simulink model "Actuators"  (Simulink 8.4)
settings: Solver=ode45  StartTime=0.0  StopTime=10.0  RelTol=1e-3
undefined symbols (not defined in the file): Ais_flgAirInjReacPumpOverride, Ais_stAirInjReacPumpMan, Apv_facAirPumpRateMan, Apv_factor, Apv_flgAirPumpRateOverride, Apv_tiPeriod_C, CDRV_E_OK_, Cov_facChOverVlvRateMan, Cov_factor, Cov_flgChOverVlvRateOverride, Cov_tiPeriod_C, Doh_OutputDiagnosisOverride, Fps_flgFuelPumpOverride, Fps_stFuelPumpMan, Icc_degIgnMan, Icc_flgIgnAngleOverride, Icc_flgIgnCutoffMan, Icc_flgIgnCutoffOverride, Icc_nrFollowUpSparks, Icc_tiDwell, Icc_tiDwellFollowUpSparks, Icc_tiOffFollowUpSparks, Ics_flgIntercoolerOverride, Ics_stIntercoolerMan, Ivc_degInjAbort, Ivc_degIntakeClose, Ivc_degOffsetInjEndSimultanInj, Ivc_flgBattDelayOverride, Ivc_flgDiagEntryCondFulfilled, Ivc_flgEndOfStartCond, Ivc_flgInjCutoff, Ivc_flgInjCutoffOverride, Ivc_flgInjTimeOverride, Ivc_flgOverrunCutoff, Ivc_flgPostInjCond, Ivc_tiBattDelayMan, Ivc_tiInjEff, Ivc_tiInjMan, Ivc_tiMinThresDeltaEffInjPeriod, Ivc_weea0, Ivc_weea1, Ivc_weea2, Lo_, Mrs_flgMainRelaisOverride, Mrs_stMainRelaisMan, Normal, OK, OpenCircuit, OverTemp, ShortToBatt, ShortToBattNEG, ShortToGnd, ShortToGndNEG, ShortToGndPOS, Str_flgStarterOverride, Str_stStarterMan, Tvc_facDutycyclePIDLimitMax, Tvc_facDutycyclePIDLimitMin, Tvc_facDutycyclePilotControlNeg, Tvc_facDutycyclePilotControlPos ... (+20)
libraries: simulink x9
(part 3 of 3)

== system Actuators/Actuators_mdl/Mrs/G1_DigOut_GetError ==
  DTC_DigOut_GetError : DataTypeConversion  OutDataTypeStr=single
  FlexECU_DevLib_FcnAPI_Wrapper_SFcn : S-Function  FunctionName=ehooks_medc17flex_devlib_basic_io_fcncall  Parameters=NoInputPorts, NoOutputPorts, InputPortDataTypes, OutputPortDataTypes, CFunctionArgTypes, CFunctionName, ChannelName  EnableBusSupport=off  mask{NoInputPorts=0, NoOutputPorts=1, InputPortDataTypes=, OutputPortDataTypes=uint8, CFunctionArgTypes=ret, CFunctionName=DevLib_DioSet_GetError, ChannelName=O_S_MRLY}
      mask prompts: NoInputPorts "Number of input ports"; NoOutputPorts "Number of output ports"; InputPortDataTypes "Input port data types"; OutputPortDataTypes "Output port data types"; CFunctionArgTypes "C function argument types"; CFunctionName "C function name"; ChannelName "Channel (pin) name"
      mask Display: disp('EHOOKS FlexECU\nDevLib Wrapper\nS-Function')
  status : Outport
  wires:
  DTC_DigOut_GetError/1 -> status/1
  FlexECU_DevLib_FcnAPI_Wrapper_SFcn/1 -> DTC_DigOut_GetError/1

== system Actuators/Actuators_mdl/Str/G1_DigOut_Ctrl ==
  state : Inport
  DTC_DigOut_ctrl : DataTypeConversion  OutDataTypeStr=uint8  RndMeth=Nearest
  DTC_Out1 : DataTypeConversion  OutDataTypeStr=boolean
  FlexECU_DevLib_FcnAPI_Wrapper_SFcn : S-Function  FunctionName=ehooks_medc17flex_devlib_basic_io_fcncall  Parameters=NoInputPorts, NoOutputPorts, InputPortDataTypes, OutputPortDataTypes, CFunctionArgTypes, CFunctionName, ChannelName  EnableBusSupport=off  mask{NoInputPorts=1, NoOutputPorts=1, InputPortDataTypes=uint8, OutputPortDataTypes=uint8, CFunctionArgTypes=ret,val, CFunctionName=DevLib_Dio_Set, ChannelName=O_S_RL34}
      mask prompts: NoInputPorts "Number of input ports"; NoOutputPorts "Number of output ports"; InputPortDataTypes "Input port data types"; OutputPortDataTypes "Output port data types"; CFunctionArgTypes "C function argument types"; CFunctionName "C function name"; ChannelName "Channel (pin) name"
      mask Display: disp('EHOOKS FlexECU\nDevLib Wrapper\nS-Function')
  status : Outport
  wires:
  DTC_DigOut_ctrl/1 -> FlexECU_DevLib_FcnAPI_Wrapper_SFcn/1
  state/1 -> DTC_DigOut_ctrl/1
  FlexECU_DevLib_FcnAPI_Wrapper_SFcn/1 -> DTC_Out1/1
  DTC_Out1/1 -> status/1

== system Actuators/Actuators_mdl/Str/G1_DigOut_GetError ==
  DTC_DigOut_GetError : DataTypeConversion  OutDataTypeStr=single
  FlexECU_DevLib_FcnAPI_Wrapper_SFcn : S-Function  FunctionName=ehooks_medc17flex_devlib_basic_io_fcncall  Parameters=NoInputPorts, NoOutputPorts, InputPortDataTypes, OutputPortDataTypes, CFunctionArgTypes, CFunctionName, ChannelName  EnableBusSupport=off  mask{NoInputPorts=0, NoOutputPorts=1, InputPortDataTypes=, OutputPortDataTypes=uint8, CFunctionArgTypes=ret, CFunctionName=DevLib_DioSet_GetError, ChannelName=O_S_RL34}
      mask prompts: NoInputPorts "Number of input ports"; NoOutputPorts "Number of output ports"; InputPortDataTypes "Input port data types"; OutputPortDataTypes "Output port data types"; CFunctionArgTypes "C function argument types"; CFunctionName "C function name"; ChannelName "Channel (pin) name"
      mask Display: disp('EHOOKS FlexECU\nDevLib Wrapper\nS-Function')
  status : Outport
  wires:
  DTC_DigOut_GetError/1 -> status/1
  FlexECU_DevLib_FcnAPI_Wrapper_SFcn/1 -> DTC_DigOut_GetError/1

== system Actuators/Actuators_mdl/Tvc/Limiter ==
  max : Inport
  in : Inport  Port=2
  min : Inport  Port=3
  Saturation Dynamic : simulink/Discontinuities/Saturation Dynamic  OutMin=[]  OutMax=[]  OutDataTypeStr=Inherit: Same as second input  OutDataType=fixdt(1, 16)  OutScaling=2^-10  DoSatur=off
  return : Outport
  wires:
  max/1 -> Saturation Dynamic/1
  in/1 -> Saturation Dynamic/2
  min/1 -> Saturation Dynamic/3
  Saturation Dynamic/1 -> return/1

== system Actuators/Actuators_mdl/Tvc/ThrottleValveControl ==
  Tvc_flgPosError : Inport
  Tvc_facThrValve : Inport  Port=2
  Tvc_facThrValveReq : Inport  Port=3
  Add : Sum  OutDataTypeStr=Inherit: Same as first input
  Constan1 : Constant  Value=0.0  OutDataTypeStr=single
  Constan2 : Constant  Value=0.01  OutDataTypeStr=single
  Constant1 : Constant  Value=Tvc_facDutycyclePilotControlPos  OutDataTypeStr=single
  Constant2 : Constant  Value=Tvc_facDutycyclePilotControlNeg  OutDataTypeStr=single
  Constant3 : Constant  Value=Tvc_flgThrValveDutycycleOverride
  Constant4 : Constant  Value=Tvc_facThrValveDutycycleMan
  Constant5 : Constant  Value=Tvc_tiTnDutycycle
  Constant6 : Constant  Value=Tvc_tiTvDutycycle
  Constant7 : Constant  Value=Tvc_facKDutycycle
  Constant8 : Constant  Value=Tvc_facDutycyclePIDLimitMax
  Constant9 : Constant  Value=Tvc_facDutycyclePIDLimitMin
  Logical Operator1 : Logic  Operator=NOT  AllPortsSameDT=off  OutDataTypeStr=boolean
  Manual Switch : ManualSwitch
  PID_Limit_AWU : Subsystem
      mask help: PID_Limit_AWU
      mask Display: image(imread('PID_Limit_AWU.jpg'))
  PID_Limit_AWU_Fcn : Subsystem
      mask help: PID_Limit_AWU_Fcn
      mask Display: image(imread('PID_Limit_AWU.jpg'))
  Relational Operator : RelationalOperator  Operator=<  OutDataTypeStr=boolean
  Subtract : Sum  Inputs=+-  OutDataTypeStr=Inherit: Same as first input
  Switch : Switch  Threshold=1
  Switch1 : Switch  Threshold=1
  Tvc_facDutycycle : Outport
  wires:
  Constant3/1 -> Switch1/2
  Constant4/1 -> Switch1/1
  Add/1 -> Switch1/3
  Constan1/1 -> Relational Operator/2
  Relational Operator/1 -> Switch/2
  Switch/1 -> Add/1
  Switch1/1 -> Tvc_facDutycycle/1
  Tvc_flgPosError/1 -> Logical Operator1/1
  Constant5/1 -> PID_Limit_AWU/1(Tn)
  Constan2/1 -> PID_Limit_AWU/3(Ta)
  Subtract/1 -> PID_Limit_AWU/5(in), PID_Limit_AWU_Fcn/1(in)
  Constant6/1 -> PID_Limit_AWU/2(Tv)
  Constant7/1 -> PID_Limit_AWU/4(Kp)
  Tvc_facThrValveReq/1 -> Subtract/2
  Tvc_facThrValve/1 -> Subtract/1, Relational Operator/1
  Constant2/1 -> Switch/1
  Constant1/1 -> Switch/3
  Logical Operator1/1 -> PID_Limit_AWU_Fcn/2(initValue), PID_Limit_AWU/6(initValue)
  Constant8/1 -> PID_Limit_AWU/7(outMax)
  Constant9/1 -> PID_Limit_AWU/8(outMin)
  PID_Limit_AWU_Fcn/1(Tvc_facDutycycleCorr) -> Manual Switch/2  "Tvc_facDutycycleCorr_Fcn"
  PID_Limit_AWU/1(Tvc_facDutycycleCorr) -> Manual Switch/1  "Tvc_facDutycycleCorr"
  Manual Switch/1 -> Add/2

== system Actuators/Actuators_mdl/Tvc/ThrottleValveOutput ==
  Tvc_flgPosError : Inport
  Tvc_facDutycycle : Inport  Port=2
  Constant1 : Constant  Value=Tvc_tiPeriod_C
  Constant3 : Constant  Value=Lo_
  Constant5 : Constant  Value=Normal
  G1_HbridgeOut_Ctrl : Subsystem  AncestorBlock=ehooks_medc17flex_G1_lib/Library Blocks/Basic_IO/Outputs/G1_HbridgeOut_Ctrl  mask{ChannelName=O_T_DC1}
      mask prompts: ChannelName "Channel name"
      mask init:
      | ehooks_medc17flex_devlib_io_block('mask_init');
      settings: AttributesFormatString=Channel name: '%<ChannelName>'
      mask TypeOptions ChannelName: <empty> | O_T_DC1 | O_T_DC2 | O_T_DC3
      mask Display: image(imread('Output_HBridge.jpg'))
  G1_Hbridge_Get_error : Subsystem  AncestorBlock=ehooks_medc17flex_G1_lib/Library Blocks/Basic_IO/Outputs/G1_Hbridge_Get_error  mask{ChannelName=O_T_DC1}
      mask prompts: ChannelName "Channel name"
      mask init:
      | ehooks_medc17flex_devlib_io_block('mask_init');
      settings: AttributesFormatString=Channel name: '%<ChannelName>'
      mask TypeOptions ChannelName: <empty> | O_T_DC1 | O_T_DC2 | O_T_DC3
      mask Display: image(imread('Output_HBridge_Diagnosis.jpg'))
  Interval Test : simulink/Logic and Bit Operations/Interval Test  IntervalClosedRight=on  uplimit=1  IntervalClosedLeft=on  lowlimit=-1  OutDataTypeStr=boolean
  Logical Operator : Logic  Operator=OR  Inputs=3  AllPortsSameDT=off  OutDataTypeStr=boolean
  Relational Operator : RelationalOperator  Operator=~=  OutDataTypeStr=boolean
  Tvc_stHBridge : Outport
  Tvc_stDiagnosis : Outport  Port=2
  wires:
  Constant1/1 -> G1_HbridgeOut_Ctrl/3(period)
  Tvc_facDutycycle/1 -> G1_HbridgeOut_Ctrl/1(dutycycle), Interval Test/1
  G1_HbridgeOut_Ctrl/1(status) -> Tvc_stHBridge/1
  Logical Operator/1 -> G1_HbridgeOut_Ctrl/2(disable)
  Interval Test/1 -> Logical Operator/1
  Constant3/1 -> G1_HbridgeOut_Ctrl/4(level)
  G1_Hbridge_Get_error/1(status) -> Tvc_stDiagnosis/1
  [Opm_idxMode_global] -> Relational Operator/1
  Constant5/1 -> Relational Operator/2
  Tvc_flgPosError/1 -> Logical Operator/2
  Relational Operator/1 -> Logical Operator/3

== system Actuators/Actuators_mdl/Tvc/ThrottleValvePosition ==
  Abs : Abs
  Add : Sum  OutDataTypeStr=Inherit: Same as first input
  Constan1 : Constant  Value=0.05  OutDataTypeStr=single
  Constant : Constant  Value=2  OutDataTypeStr=single
  Divide : Product  Inputs=*/  OutDataTypeStr=Inherit: Same as first input
  G1_ADC_Input_Receive : Subsystem  AncestorBlock=ehooks_medc17flex_G1_lib/Library Blocks/Basic_IO/Inputs/G1_ADC_Input_Receive  mask{ChannelName=I_A_AN01}
      mask prompts: ChannelName "Channel name"
      mask init:
      | ehooks_medc17flex_devlib_io_block('mask_init');
      settings: AttributesFormatString=Channel name: '%<ChannelName>'
      mask TypeOptions ChannelName: <empty> | I_A_AN01 | I_A_AN02 | I_A_AN03 | I_A_AN05 | I_A_AN06 | I_A_AN07 | I_A_AN08 | I_A_AN10 | I_A_AN11 | I_A_AN12 | I_A_AN13 | I_A_AN14 | I_A_AN15 | I_A_AN16 | I_A_AN17 | I_A_AN18 | I_A_AN19 | I_A_AN20 | I_A_AN21 | I_A_AN23 | I_A_AN32 | I_A_AN35 | I_A_AN36 | I_A_AN37 | I_A_AN39 | I_A_AN100 | I_A_AN101 | I_A_AN103 | I_A_AN104 | I_A_AN105 | I_A_AN106
      mask Display: image(imread('Input_Analog.jpg'))
  G1_ADC_Input_Receive1 : Subsystem  AncestorBlock=ehooks_medc17flex_G1_lib/Library Blocks/Basic_IO/Inputs/G1_ADC_Input_Receive  mask{ChannelName=I_A_AN02}
      mask prompts: ChannelName "Channel name"
      mask init:
      | ehooks_medc17flex_devlib_io_block('mask_init');
      settings: AttributesFormatString=Channel name: '%<ChannelName>'
      mask TypeOptions ChannelName: <empty> | I_A_AN01 | I_A_AN02 | I_A_AN03 | I_A_AN05 | I_A_AN06 | I_A_AN07 | I_A_AN08 | I_A_AN10 | I_A_AN11 | I_A_AN12 | I_A_AN13 | I_A_AN14 | I_A_AN15 | I_A_AN16 | I_A_AN17 | I_A_AN18 | I_A_AN19 | I_A_AN20 | I_A_AN21 | I_A_AN23 | I_A_AN32 | I_A_AN35 | I_A_AN36 | I_A_AN37 | I_A_AN39 | I_A_AN100 | I_A_AN101 | I_A_AN103 | I_A_AN104 | I_A_AN105 | I_A_AN106
      mask Display: image(imread('Input_Analog.jpg'))
  Interval Test : simulink/Logic and Bit Operations/Interval Test  IntervalClosedRight=on  uplimit=Tvc_uSensMaxValid  IntervalClosedLeft=on  lowlimit=Tvc_uSensMinValid  OutDataTypeStr=boolean
  Interval Test1 : simulink/Logic and Bit Operations/Interval Test  IntervalClosedRight=on  uplimit=Tvc_uSensMaxValid  IntervalClosedLeft=on  lowlimit=Tvc_uSensMinValid  OutDataTypeStr=boolean
  Logical Operator{,1..3} (4 alike) : Logic  Operator=NOT  AllPortsSameDT=off  OutDataTypeStr=boolean
  Logical Operator4 : Logic  Operator=OR  Inputs=5  AllPortsSameDT=off  OutDataTypeStr=boolean
  Relational Oprator : RelationalOperator  Operator=>  OutDataTypeStr=boolean
  Subtract : Sum  Inputs=+-  OutDataTypeStr=Inherit: Same as first input
  Tvc_uSens2facThrValve1_CUR : Lookup_n-D  NumberOfTableDimensions=1  BreakpointsForDimension1=[1:3]  Table=[1 3 6]  ExtrapMethod=Clip  OutDataTypeStr=Inherit: Inherit from 'Table data'  InputSameDT=on
  Tvc_uSens2facThrValve2_CUR : Lookup_n-D  NumberOfTableDimensions=1  BreakpointsForDimension1=[1:3]  Table=[1 2 7]  ExtrapMethod=Clip  OutDataTypeStr=Inherit: Inherit from 'Table data'  InputSameDT=on
  Tvc_flgPosError : Outport
  Tvc_facThrValve : Outport  Port=2
  wires:
  G1_ADC_Input_Receive/1(status) -> Logical Operator/1  "Tvc_stIO1"
  G1_ADC_Input_Receive/2(uRaw) -> Tvc_uSens2facThrValve1_CUR/1, Interval Test/1  "Tvc_uSens1"
  G1_ADC_Input_Receive1/1(status) -> Logical Operator2/1  "Tvc_stIO2"
  G1_ADC_Input_Receive1/2(uRaw) -> Tvc_uSens2facThrValve2_CUR/1, Interval Test1/1  "Tvc_uSens2"
  Interval Test/1 -> Logical Operator1/1
  Interval Test1/1 -> Logical Operator3/1
  Tvc_uSens2facThrValve1_CUR/1 -> Add/1, Subtract/1  "Tvc_facThrValve1"
  Tvc_uSens2facThrValve2_CUR/1 -> Add/2, Subtract/2  "Tvc_facThrValve2"
  Add/1 -> Divide/1
  Constant/1 -> Divide/2
  Subtract/1 -> Abs/1
  Abs/1 -> Relational Oprator/1
  Constan1/1 -> Relational Oprator/2
  Logical Operator4/1 -> Tvc_flgPosError/1
  Logical Operator/1 -> Logical Operator4/1
  Logical Operator1/1 -> Logical Operator4/2
  Logical Operator2/1 -> Logical Operator4/3
  Logical Operator3/1 -> Logical Operator4/4
  Relational Oprator/1 -> Logical Operator4/5
  Divide/1 -> Tvc_facThrValve/1

== system Actuators/Actuators_mdl/Wcs/G1_DigOut_Ctrl ==
  state : Inport
  DTC_DigOut_ctrl : DataTypeConversion  OutDataTypeStr=uint8  RndMeth=Nearest
  DTC_Out1 : DataTypeConversion  OutDataTypeStr=boolean
  FlexECU_DevLib_FcnAPI_Wrapper_SFcn : S-Function  FunctionName=ehooks_medc17flex_devlib_basic_io_fcncall  Parameters=NoInputPorts, NoOutputPorts, InputPortDataTypes, OutputPortDataTypes, CFunctionArgTypes, CFunctionName, ChannelName  EnableBusSupport=off  mask{NoInputPorts=1, NoOutputPorts=1, InputPortDataTypes=uint8, OutputPortDataTypes=uint8, CFunctionArgTypes=ret,val, CFunctionName=DevLib_Dio_Set, ChannelName=O_S_RL14}
      mask prompts: NoInputPorts "Number of input ports"; NoOutputPorts "Number of output ports"; InputPortDataTypes "Input port data types"; OutputPortDataTypes "Output port data types"; CFunctionArgTypes "C function argument types"; CFunctionName "C function name"; ChannelName "Channel (pin) name"
      mask Display: disp('EHOOKS FlexECU\nDevLib Wrapper\nS-Function')
  status : Outport
  wires:
  DTC_DigOut_ctrl/1 -> FlexECU_DevLib_FcnAPI_Wrapper_SFcn/1
  state/1 -> DTC_DigOut_ctrl/1
  FlexECU_DevLib_FcnAPI_Wrapper_SFcn/1 -> DTC_Out1/1
  DTC_Out1/1 -> status/1

== system Actuators/Actuators_mdl/Wcs/G1_DigOut_GetError ==
  DTC_DigOut_GetError : DataTypeConversion  OutDataTypeStr=single
  FlexECU_DevLib_FcnAPI_Wrapper_SFcn : S-Function  FunctionName=ehooks_medc17flex_devlib_basic_io_fcncall  Parameters=NoInputPorts, NoOutputPorts, InputPortDataTypes, OutputPortDataTypes, CFunctionArgTypes, CFunctionName, ChannelName  EnableBusSupport=off  mask{NoInputPorts=0, NoOutputPorts=1, InputPortDataTypes=, OutputPortDataTypes=uint8, CFunctionArgTypes=ret, CFunctionName=DevLib_DioSet_GetError, ChannelName=O_S_RL14}
      mask prompts: NoInputPorts "Number of input ports"; NoOutputPorts "Number of output ports"; InputPortDataTypes "Input port data types"; OutputPortDataTypes "Output port data types"; CFunctionArgTypes "C function argument types"; CFunctionName "C function name"; ChannelName "Channel (pin) name"
      mask Display: disp('EHOOKS FlexECU\nDevLib Wrapper\nS-Function')
  status : Outport
  wires:
  DTC_DigOut_GetError/1 -> status/1
  FlexECU_DevLib_FcnAPI_Wrapper_SFcn/1 -> DTC_DigOut_GetError/1

== system Actuators/Actuators_mdl/Wcs/Hysteresis_Delta_RSP ==
  in : Inport
  Relay : Relay  OnSwitchValue=Wcs_atCoolantMax  OffSwitchValue=Wcs_atCoolantMax-Wcs_atCoolantHyst  OutDataTypeStr=Inherit: Inherit via back propagation
  return : Outport
  wires:
  in/1 -> Relay/1
  Relay/1 -> return/1

== system Actuators/Actuators_mdl/Wgc/G1_PWM_Output_Ctrl ==
  dutycycle : Inport
  period : Inport  Port=2
  factor : Inport  Port=3
  level : Inport  Port=4
  DTC_PwmOut_DutyCycle : DataTypeConversion  OutDataTypeStr=int16  RndMeth=Nearest
  DTC_PwmOut_ErrorInfo : DataTypeConversion  OutDataTypeStr=boolean
  DTC_PwmOut_Level : DataTypeConversion  OutDataTypeStr=int16  RndMeth=Nearest
  DTC_PwmOut_Period : DataTypeConversion  OutDataTypeStr=int16  RndMeth=Nearest
  DTC_PwmOut_Period1 : DataTypeConversion  OutDataTypeStr=uint8  RndMeth=Nearest
  FlexECU_DevLib_FcnAPI_Wrapper_SFcn : S-Function  FunctionName=ehooks_medc17flex_devlib_basic_io_fcncall  Parameters=NoInputPorts, NoOutputPorts, InputPortDataTypes, OutputPortDataTypes, CFunctionArgTypes, CFunctionName, ChannelName  EnableBusSupport=off  mask{NoInputPorts=4, NoOutputPorts=1, InputPortDataTypes=int16,int16, int16, uint8, OutputPortDataTypes=uint8, CFunctionArgTypes=ret,val,val,val,val, CFunctionName=DevLib_Pwm_Out, ChannelName=O_T_RL22}
      mask prompts: NoInputPorts "Number of input ports"; NoOutputPorts "Number of output ports"; InputPortDataTypes "Input port data types"; OutputPortDataTypes "Output port data types"; CFunctionArgTypes "C function argument types"; CFunctionName "C function name"; ChannelName "Channel (pin) name"
      mask Display: disp('EHOOKS FlexECU\nDevLib Wrapper\nS-Function')
  Gain : Gain  Gain=100
  status : Outport
  wires:
  Gain/1 -> DTC_PwmOut_DutyCycle/1
  dutycycle/1 -> Gain/1
  level/1 -> DTC_PwmOut_Period1/1
  DTC_PwmOut_Period1/1 -> FlexECU_DevLib_FcnAPI_Wrapper_SFcn/4
  FlexECU_DevLib_FcnAPI_Wrapper_SFcn/1 -> DTC_PwmOut_ErrorInfo/1
  period/1 -> DTC_PwmOut_Period/1
  factor/1 -> DTC_PwmOut_Level/1
  DTC_PwmOut_DutyCycle/1 -> FlexECU_DevLib_FcnAPI_Wrapper_SFcn/1
  DTC_PwmOut_Period/1 -> FlexECU_DevLib_FcnAPI_Wrapper_SFcn/2
  DTC_PwmOut_Level/1 -> FlexECU_DevLib_FcnAPI_Wrapper_SFcn/3
  DTC_PwmOut_ErrorInfo/1 -> status/1

== system Actuators/Actuators_mdl/Wgc/G1_PwmOut_Get_error ==
  DTC_PwmOut_GetError : DataTypeConversion  OutDataTypeStr=single
  FlexECU_DevLib_FcnAPI_Wrapper_SFcn : S-Function  FunctionName=ehooks_medc17flex_devlib_basic_io_fcncall  Parameters=NoInputPorts, NoOutputPorts, InputPortDataTypes, OutputPortDataTypes, CFunctionArgTypes, CFunctionName, ChannelName  EnableBusSupport=off  mask{NoInputPorts=0, NoOutputPorts=1, InputPortDataTypes=, OutputPortDataTypes=uint8, CFunctionArgTypes=ret, CFunctionName=DevLib_PwmOut_GetError, ChannelName=O_T_RL22}
      mask prompts: NoInputPorts "Number of input ports"; NoOutputPorts "Number of output ports"; InputPortDataTypes "Input port data types"; OutputPortDataTypes "Output port data types"; CFunctionArgTypes "C function argument types"; CFunctionName "C function name"; ChannelName "Channel (pin) name"
      mask Display: disp('EHOOKS FlexECU\nDevLib Wrapper\nS-Function')
  status : Outport
  wires:
  DTC_PwmOut_GetError/1 -> status/1
  FlexECU_DevLib_FcnAPI_Wrapper_SFcn/1 -> DTC_PwmOut_GetError/1

== system Actuators/Actuators_mdl/Ivc/Ivc/G1_InjVlvPFI_SetParam ==
  te_i : Inport
  tez_i1 : Inport  Port=2
  tez_i2 : Inport  Port=3
  tez_i3 : Inport  Port=4
  tez_i4 : Inport  Port=5
  tez_i5 : Inport  Port=6
  tez_i6 : Inport  Port=7
  tez_i7 : Inport  Port=8
  tez_i8 : Inport  Port=9
  dtemnkt_w : Inport  Port=10
  tvub_w : Inport  Port=11
  B_nsp : Inport  Port=12
  B_stendes : Inport  Port=13
  evz_austot : Inport  Port=14
  wea : Inport  Port=15
  weea_1 : Inport  Port=16
  weea_2 : Inport  Port=17
  weea_3 : Inport  Port=18
  weestim : Inport  Port=19
  wes : Inport  Port=20
  DTC_PFI_B_nsp : DataTypeConversion  OutDataTypeStr=uint8  RndMeth=Nearest
  DTC_PFI_B_stendes : DataTypeConversion  OutDataTypeStr=uint8  RndMeth=Nearest
  DTC_PFI_B_weea_1 : DataTypeConversion  OutDataTypeStr=uint8  RndMeth=Nearest
  DTC_PFI_B_weea_2 : DataTypeConversion  OutDataTypeStr=uint8
  DTC_PFI_B_weea_3 : DataTypeConversion  OutDataTypeStr=uint8  RndMeth=Nearest
  DTC_PFI_B_weestsim : DataTypeConversion  OutDataTypeStr=uint8  RndMeth=Nearest
  DTC_PFI_CdrvError : DataTypeConversion  OutDataTypeStr=single
  DTC_PFI_dtemnkt_w : DataTypeConversion  OutDataTypeStr=uint16  RndMeth=Nearest
  DTC_PFI_evz_austot : DataTypeConversion  OutDataTypeStr=uint8  RndMeth=Nearest
  DTC_PFI_te_l : DataTypeConversion  OutDataTypeStr=uint32  RndMeth=Nearest
  DTC_PFI_tez_8 : DataTypeConversion  OutDataTypeStr=uint32  RndMeth=Nearest
  DTC_PFI_tez_i{1..7} (7 alike) : DataTypeConversion  OutDataTypeStr=uint32  RndMeth=Nearest
  DTC_PFI_tvub_w : DataTypeConversion  OutDataTypeStr=uint16  RndMeth=Nearest
  DTC_PFI_wea : DataTypeConversion  OutDataTypeStr=uint8  RndMeth=Nearest
  DTC_PFI_wes : DataTypeConversion  OutDataTypeStr=uint8  RndMeth=Nearest
  FlexECU_SFcn_PFI_inj : S-Function  FunctionName=ehooks_medc17flex_devlib_ign_struct_fcncall  Parameters=NoInputPorts, NoOutputPorts, InputPortDataTypes, OutputPortDataTypes, CFunctionArgTypes, CFunctionName, StructMemberNames, StructTypeName, InputPortDataWidths, OutputPortDataWidths  EnableBusSupport=off  mask{NoInputPorts=11, NoOutputPorts=1, InputPortDataTypes=uint32, uint32, uint16, uint16,uint8,uint8,uint8,uint8,uint8,uint8,uint8, OutputPortDataTypes=uint8, CFunctionArgTypes=ret,val, refin, val,val,val,val,val, val, refin, val, val, CFunctionName=InjVlvPfi_SetParam, StructMemberNames=te_l,  tez_l, dtemnkt_w, tvub_w, B_nsp, B_stendes, evz_austot, wea, weea, weestsim, wes, StructTypeName=InjVlvPfiInterface_type, InputPortDataWidths=1,8,1,1,1,1,1,1,3,1,1, OutputPortDataWidths=1}
      mask prompts: NoInputPorts "Number of input ports"; NoOutputPorts "Number of output ports"; InputPortDataTypes "Input port data types"; OutputPortDataTypes "Output port data types"; CFunctionArgTypes "C function argument types"; CFunctionName "C function name"; StructMemberNames "Structure member names"; StructTypeName "Structure type name"; InputPortDataWidths "Input port widths"; OutputPortDataWidths "Output port widths"
      mask Display: disp('EHOOKS FlexECU\nDevLib Wrapper\nS-Function')
  Mux : Mux  Inputs=8
  Mux1 : Mux  Inputs=3
  Cdrv_Error : Outport
  wires:
  DTC_PFI_CdrvError/1 -> Cdrv_Error/1
  FlexECU_SFcn_PFI_inj/1 -> DTC_PFI_CdrvError/1
  DTC_PFI_B_stendes/1 -> FlexECU_SFcn_PFI_inj/6
  B_stendes/1 -> DTC_PFI_B_stendes/1
  DTC_PFI_B_nsp/1 -> FlexECU_SFcn_PFI_inj/5
  B_nsp/1 -> DTC_PFI_B_nsp/1
  DTC_PFI_tvub_w/1 -> FlexECU_SFcn_PFI_inj/4
  tvub_w/1 -> DTC_PFI_tvub_w/1
  DTC_PFI_dtemnkt_w/1 -> FlexECU_SFcn_PFI_inj/3
  dtemnkt_w/1 -> DTC_PFI_dtemnkt_w/1
  te_i/1 -> DTC_PFI_te_l/1
  DTC_PFI_evz_austot/1 -> FlexECU_SFcn_PFI_inj/7
  DTC_PFI_wea/1 -> FlexECU_SFcn_PFI_inj/8
  DTC_PFI_B_weestsim/1 -> FlexECU_SFcn_PFI_inj/10
  DTC_PFI_wes/1 -> FlexECU_SFcn_PFI_inj/11
  evz_austot/1 -> DTC_PFI_evz_austot/1
  wea/1 -> DTC_PFI_wea/1
  weea_1/1 -> DTC_PFI_B_weea_1/1
  weestim/1 -> DTC_PFI_B_weestsim/1
  wes/1 -> DTC_PFI_wes/1
  DTC_PFI_te_l/1 -> FlexECU_SFcn_PFI_inj/1
  tez_i1/1 -> DTC_PFI_tez_i1/1
  tez_i2/1 -> DTC_PFI_tez_i2/1
  tez_i3/1 -> DTC_PFI_tez_i3/1
  tez_i4/1 -> DTC_PFI_tez_i4/1
  tez_i5/1 -> DTC_PFI_tez_i5/1
  tez_i6/1 -> DTC_PFI_tez_i6/1
  tez_i7/1 -> DTC_PFI_tez_i7/1
  tez_i8/1 -> DTC_PFI_tez_8/1
  DTC_PFI_tez_i1/1 -> Mux/1
  DTC_PFI_tez_i2/1 -> Mux/2
  DTC_PFI_tez_i3/1 -> Mux/3
  DTC_PFI_tez_i4/1 -> Mux/4
  DTC_PFI_tez_i5/1 -> Mux/5
  DTC_PFI_tez_i6/1 -> Mux/6
  DTC_PFI_tez_i7/1 -> Mux/7
  DTC_PFI_tez_8/1 -> Mux/8
  Mux/1 -> FlexECU_SFcn_PFI_inj/2  "tez_xxx"
  weea_2/1 -> DTC_PFI_B_weea_2/1
  weea_3/1 -> DTC_PFI_B_weea_3/1
  DTC_PFI_B_weea_1/1 -> Mux1/1
  DTC_PFI_B_weea_2/1 -> Mux1/2
  DTC_PFI_B_weea_3/1 -> Mux1/3
  Mux1/1 -> FlexECU_SFcn_PFI_inj/9  "weea_xxx"

== system Actuators/Actuators_mdl/Ivc/Ivc_Diag/G1_Inj_Set_DEVE_forPFI ==
  B_desee : Inport
  B_sa : Inport  Port=2
  DTC_PFI_DEVE_Bdesee : DataTypeConversion  OutDataTypeStr=uint8  RndMeth=Nearest
  DTC_PFI_DEVE_Bsa : DataTypeConversion  OutDataTypeStr=uint8  RndMeth=Nearest
  DTC_PFI_DEVE_Bsa1 : DataTypeConversion  OutDataTypeStr=single
  FlexECU_SFcn_PFI_inj : S-Function  FunctionName=ehooks_medc17flex_devlib_ign_struct_fcncall  Parameters=NoInputPorts, NoOutputPorts, InputPortDataTypes, OutputPortDataTypes, CFunctionArgTypes, CFunctionName, StructMemberNames, StructTypeName, InputPortDataWidths, OutputPortDataWidths  EnableBusSupport=off  mask{NoInputPorts=2, NoOutputPorts=1, InputPortDataTypes=uint8,uint8, OutputPortDataTypes=uint8, CFunctionArgTypes=ret, val, val, CFunctionName=InjVlvDeve_SetParam, StructMemberNames=B_desee, B_sa, StructTypeName=InjVlvDeveInterface_type, InputPortDataWidths=1,1, OutputPortDataWidths=1}
      mask prompts: NoInputPorts "Number of input ports"; NoOutputPorts "Number of output ports"; InputPortDataTypes "Input port data types"; OutputPortDataTypes "Output port data types"; CFunctionArgTypes "C function argument types"; CFunctionName "C function name"; StructMemberNames "Structure member names"; StructTypeName "Structure type name"; InputPortDataWidths "Input port widths"; OutputPortDataWidths "Output port widths"
      mask Display: disp('EHOOKS FlexECU\nDevLib Wrapper\nS-Function')
  Cdrv_Error : Outport
  wires:
  DTC_PFI_DEVE_Bsa/1 -> FlexECU_SFcn_PFI_inj/2
  B_sa/1 -> DTC_PFI_DEVE_Bsa/1
  B_desee/1 -> DTC_PFI_DEVE_Bdesee/1
  DTC_PFI_DEVE_Bdesee/1 -> FlexECU_SFcn_PFI_inj/1
  FlexECU_SFcn_PFI_inj/1 -> DTC_PFI_DEVE_Bsa1/1
  DTC_PFI_DEVE_Bsa1/1 -> Cdrv_Error/1

== system Actuators/Actuators_mdl/Tvc/ThrottleValveControl/PID_Limit_AWU ==
  Tn : Inport
  Tv : Inport  Port=2
  Ta : Inport  Port=3
  Kp : Inport  Port=4
  in : Inport  Port=5
  initValue : Inport  Port=6
  outMax : Inport  Port=7
  outMin : Inport  Port=8
  Add : Sum  OutDataTypeStr=Inherit: Same as first input
  Add1 : Sum  Inputs=+++  OutDataTypeStr=Inherit: Same as first input
  Constant1 : Constant  Value=0.0  OutDataTypeStr=single
  Constant10 : Constant  Value=0.0  OutDataTypeStr=single
  Divide : Product  Inputs=*/  OutDataTypeStr=Inherit: Same as first input
  Divide1 : Product  Inputs=*/  OutDataTypeStr=Inherit: Same as first input
  Interval Test : simulink/Logic and Bit Operations/Interval Test  IntervalClosedRight=on  uplimit=Tvc_facDutycyclePIDLimitMax  IntervalClosedLeft=on  lowlimit=Tvc_facDutycyclePIDLimitMin  LogicOutDataTypeMode=boolean
  Limiter : Subsystem
      mask help: Limiter
      mask Display: image(imread('Limiter.jpg'))
  Product : Product  OutDataTypeStr=Inherit: Same as first input
  Product1 : Product  OutDataTypeStr=Inherit: Same as first input
  Product2 : Product  Inputs=3  OutDataTypeStr=Inherit: Same as first input
  Product3 : Product  OutDataTypeStr=Inherit: Same as first input
  Subtract : Sum  Inputs=+-  OutDataTypeStr=Inherit: Same as first input
  Switch1 : Switch  Threshold=1
  Switch2 : Switch  Threshold=1
  Unit Delay1 : UnitDelay  SampleTime=-1
  Unit Delay2 : UnitDelay  SampleTime=-1
  Tvc_facDutycycleCorr : Outport
  wires:
  Constant10/1 -> Switch2/3
  Product2/1 -> Switch2/1
  Interval Test/1 -> Switch2/2
  Unit Delay2/1 -> Add/2, Add1/2
  Add/1 -> Unit Delay2/1
  Unit Delay1/1 -> Subtract/2
  Kp/1 -> Product/1, Product3/2, Divide1/1
  Tv/1 -> Product/2
  Product/1 -> Divide/1
  Ta/1 -> Product2/1, Divide/2
  Divide/1 -> Product1/1
  Tn/1 -> Divide1/2
  in/1 -> Product2/2, Product3/1, Subtract/1, Unit Delay1/1  "inOLD"
  Divide1/1 -> Product2/3
  Subtract/1 -> Product1/2
  Switch2/1 -> Add/1
  Product3/1 -> Add1/3
  Product1/1 -> Add1/1
  Add1/1 -> Limiter/2(in), Interval Test/1
  outMin/1 -> Limiter/3(min)
  outMax/1 -> Limiter/1(max)
  Constant1/1 -> Switch1/3
  initValue/1 -> Switch1/2
  Switch1/1 -> Tvc_facDutycycleCorr/1
  Limiter/1(return) -> Switch1/1

== system Actuators/Actuators_mdl/Tvc/ThrottleValveControl/PID_Limit_AWU_Fcn ==
  in : Inport
  initValue : Inport  Port=2
  Constant1 : Constant  Value=0.0  OutDataTypeStr=single
  Discrete PID Controller : simulink/Continuous/PID Controller  Controller=PID  TimeDomain=Discrete-time  SampleTime=-1  IntegratorMethod=Forward Euler  FilterMethod=Forward Euler  Form=Parallel  P=Tvc_facKDutycycle  I=Tvc_facKDutycycle/Tvc_tiTnDutycycle  D=Tvc_facKDutycycle*Tvc_tiTvDutycycle  N=Tvc_facKDutycycle*Tvc_tiTvDutycycle/0.01  InitialConditionSource=internal  InitialConditionForIntegrator=0  InitialConditionForFilter=0  ExternalReset=none  LimitOutput=on  UpperSaturationLimit=Tvc_facDutycyclePIDLimitMax  LowerSaturationLimit=Tvc_facDutycyclePIDLimitMin  LinearizeAsGain=off  AntiWindupMode=none  Kb=1  TrackingMode=off  Kt=1  PParamMin=[]  PParamMax=[]  IParamMin=[]  IParamMax=[]  DParamMin=[]  DParamMax=[]  NParamMin=[]  NParamMax=[]  KbParamMin=[]  KbParamMax=[]  KtParamMin=[]  KtParamMax=[]  POutMin=[]  POutMax=[]  IOutMin=[]  IOutMax=[]  DOutMin=[]  DOutMax=[]  NOutMin=[]  NOutMax=[]  KbOutMin=[]  KbOutMax=[]  KtOutMin=[]  KtOutMax=[]  IntegratorOutMin=[]  IntegratorOutMax=[]  FilterOutMin=[]  FilterOutMax=[]  SumOutMin=[]  SumOutMax=[]  SumI1OutMin=[]  SumI1OutMax=[]  SumI2OutMin=[]  SumI2OutMax=[]  SumI3OutMin=[]  SumI3OutMax=[]  SumDOutMin=[]  SumDOutMax=[]  SaturationOutMin=[]  SaturationOutMax=[]  IntegratorContinuousStateAttributes=''  IntegratorStateMustResolveToSignalObject=off  IntegratorRTWStateStorageClass=Auto  FilterContinuousStateAttributes=''  FilterStateMustResolveToSignalObject=off  FilterRTWStateStorageClass=Auto
  Switch1 : Switch  Threshold=1
  Tvc_facDutycycleCorr : Outport
  wires:
  Switch1/1 -> Tvc_facDutycycleCorr/1
  initValue/1 -> Switch1/2
  Constant1/1 -> Switch1/3
  in/1 -> Discrete PID Controller/1  "inOLD"
  Discrete PID Controller/1 -> Switch1/1

== system Actuators/Actuators_mdl/Tvc/ThrottleValveOutput/G1_HbridgeOut_Ctrl ==
  dutycycle : Inport
  disable : Inport  Port=2
  period : Inport  Port=3
  level : Inport  Port=4
  DTC_HB_Disable : DataTypeConversion  OutDataTypeStr=uint8  RndMeth=Nearest
  DTC_HB_DutyCycle : DataTypeConversion  OutDataTypeStr=int16  RndMeth=Nearest
  DTC_HB_ErrorInfo : DataTypeConversion  OutMin=0.0  OutMax=1.0  OutDataTypeStr=boolean
  DTC_HB_Level : DataTypeConversion  OutDataTypeStr=uint8  RndMeth=Nearest
  DTC_HB_Period : DataTypeConversion  OutDataTypeStr=int16  RndMeth=Nearest
  FlexECU_DevLib_FcnAPI_Wrapper_SFcn : S-Function  FunctionName=ehooks_medc17flex_devlib_basic_io_fcncall  Parameters=NoInputPorts, NoOutputPorts, InputPortDataTypes, OutputPortDataTypes, CFunctionArgTypes, CFunctionName, ChannelName  EnableBusSupport=off  mask{NoInputPorts=4, NoOutputPorts=1, InputPortDataTypes=int16,uint8,int16,uint8, OutputPortDataTypes=uint8, CFunctionArgTypes=ret,val,val,val, val, CFunctionName=DevLib_HBridge_Out, ChannelName=O_T_DC1}
      mask prompts: NoInputPorts "Number of input ports"; NoOutputPorts "Number of output ports"; InputPortDataTypes "Input port data types"; OutputPortDataTypes "Output port data types"; CFunctionArgTypes "C function argument types"; CFunctionName "C function name"; ChannelName "Channel (pin) name"
      mask Display: disp('EHOOKS FlexECU\nDevLib Wrapper\nS-Function')
  Gain : Gain  Gain=100
  status : Outport
  wires:
  Gain/1 -> DTC_HB_DutyCycle/1
  disable/1 -> DTC_HB_Disable/1
  DTC_HB_Disable/1 -> FlexECU_DevLib_FcnAPI_Wrapper_SFcn/2
  DTC_HB_Level/1 -> FlexECU_DevLib_FcnAPI_Wrapper_SFcn/4
  DTC_HB_Period/1 -> FlexECU_DevLib_FcnAPI_Wrapper_SFcn/3
  DTC_HB_ErrorInfo/1 -> status/1
  DTC_HB_DutyCycle/1 -> FlexECU_DevLib_FcnAPI_Wrapper_SFcn/1
  level/1 -> DTC_HB_Level/1
  period/1 -> DTC_HB_Period/1
  FlexECU_DevLib_FcnAPI_Wrapper_SFcn/1 -> DTC_HB_ErrorInfo/1
  dutycycle/1 -> Gain/1

== system Actuators/Actuators_mdl/Tvc/ThrottleValveOutput/G1_Hbridge_Get_error ==
  DTC_HB_GetError : DataTypeConversion  OutMin=0  OutMax=7  OutDataTypeStr=single
  FlexECU_DevLib_FcnAPI_Wrapper_SFcn : S-Function  FunctionName=ehooks_medc17flex_devlib_basic_io_fcncall  Parameters=NoInputPorts, NoOutputPorts, InputPortDataTypes, OutputPortDataTypes, CFunctionArgTypes, CFunctionName, ChannelName  EnableBusSupport=off  mask{NoInputPorts=0, NoOutputPorts=1, InputPortDataTypes=, OutputPortDataTypes=uint8, CFunctionArgTypes=ret, CFunctionName=DevLib_HBridge_GetError, ChannelName=O_T_DC1}
      mask prompts: NoInputPorts "Number of input ports"; NoOutputPorts "Number of output ports"; InputPortDataTypes "Input port data types"; OutputPortDataTypes "Output port data types"; CFunctionArgTypes "C function argument types"; CFunctionName "C function name"; ChannelName "Channel (pin) name"
      mask Display: disp('EHOOKS FlexECU\nDevLib Wrapper\nS-Function')
  status : Outport
  wires:
  FlexECU_DevLib_FcnAPI_Wrapper_SFcn/1 -> DTC_HB_GetError/1
  DTC_HB_GetError/1 -> status/1

== system Actuators/Actuators_mdl/Tvc/ThrottleValvePosition/G1_ADC_Input_Receive ==
  Data Type Conversion : DataTypeConversion  OutMin=0.0  OutMax=5.0  OutDataTypeStr=single
  Data Type Conversion1 : DataTypeConversion  OutMin=0.0  OutMax=1.0  OutDataTypeStr=boolean
  FlexECU_DevLib_FcnAPI_Wrapper_SFcn : S-Function  FunctionName=ehooks_medc17flex_devlib_basic_io_fcncall  Parameters=NoInputPorts, NoOutputPorts, InputPortDataTypes, OutputPortDataTypes, CFunctionArgTypes, CFunctionName, ChannelName  EnableBusSupport=off  mask{NoInputPorts=0, NoOutputPorts=2, InputPortDataTypes=, OutputPortDataTypes=uint8,int16, CFunctionArgTypes=ret,ref, CFunctionName=DevLib_Adc_Get, ChannelName=I_A_AN01}
      mask prompts: NoInputPorts "Number of input ports"; NoOutputPorts "Number of output ports"; InputPortDataTypes "Input port data types"; OutputPortDataTypes "Output port data types"; CFunctionArgTypes "C function argument types"; CFunctionName "C function name"; ChannelName "Channel (pin) name"
      mask Display: disp('EHOOKS FlexECU\nDevLib Wrapper\nS-Function')
  Gain : Gain  Gain=5/1023  OutDataTypeStr=Inherit: Same as input
  status : Outport
  uRaw : Outport  Port=2
  wires:
  Data Type Conversion1/1 -> status/1
  Data Type Conversion/1 -> Gain/1
  FlexECU_DevLib_FcnAPI_Wrapper_SFcn/2 -> Data Type Conversion/1
  FlexECU_DevLib_FcnAPI_Wrapper_SFcn/1 -> Data Type Conversion1/1
  Gain/1 -> uRaw/1

== system Actuators/Actuators_mdl/Tvc/ThrottleValvePosition/G1_ADC_Input_Receive1 ==
  Data Type Conversion : DataTypeConversion  OutMin=0.0  OutMax=5.0  OutDataTypeStr=single
  Data Type Conversion1 : DataTypeConversion  OutMin=0.0  OutMax=1.0  OutDataTypeStr=boolean
  FlexECU_DevLib_FcnAPI_Wrapper_SFcn : S-Function  FunctionName=ehooks_medc17flex_devlib_basic_io_fcncall  Parameters=NoInputPorts, NoOutputPorts, InputPortDataTypes, OutputPortDataTypes, CFunctionArgTypes, CFunctionName, ChannelName  EnableBusSupport=off  mask{NoInputPorts=0, NoOutputPorts=2, InputPortDataTypes=, OutputPortDataTypes=uint8,int16, CFunctionArgTypes=ret,ref, CFunctionName=DevLib_Adc_Get, ChannelName=I_A_AN02}
      mask prompts: NoInputPorts "Number of input ports"; NoOutputPorts "Number of output ports"; InputPortDataTypes "Input port data types"; OutputPortDataTypes "Output port data types"; CFunctionArgTypes "C function argument types"; CFunctionName "C function name"; ChannelName "Channel (pin) name"
      mask Display: disp('EHOOKS FlexECU\nDevLib Wrapper\nS-Function')
  Gain : Gain  Gain=5/1023  OutDataTypeStr=Inherit: Same as input
  status : Outport
  uRaw : Outport  Port=2
  wires:
  Data Type Conversion1/1 -> status/1
  Data Type Conversion/1 -> Gain/1
  FlexECU_DevLib_FcnAPI_Wrapper_SFcn/2 -> Data Type Conversion/1
  FlexECU_DevLib_FcnAPI_Wrapper_SFcn/1 -> Data Type Conversion1/1
  Gain/1 -> uRaw/1

== system Actuators/Actuators_mdl/Tvc/ThrottleValveControl/PID_Limit_AWU/Limiter ==
  max : Inport
  in : Inport  Port=2
  min : Inport  Port=3
  Saturation Dynamic : simulink/Discontinuities/Saturation Dynamic  OutMin=[]  OutMax=[]  OutDataTypeStr=Inherit: Same as second input  OutDataType=fixdt(1, 16)  OutScaling=2^-10  DoSatur=off
  return : Outport
  wires:
  max/1 -> Saturation Dynamic/1
  in/1 -> Saturation Dynamic/2
  min/1 -> Saturation Dynamic/3
  Saturation Dynamic/1 -> return/1
